simulink model "simplified_model"  (R2018b)
settings: Solver=VariableStepAuto  StartTime=0.0  StopTime=20  RelTol=1e-3
settings Model: Creator=dylan  LastModifiedBy=dylan

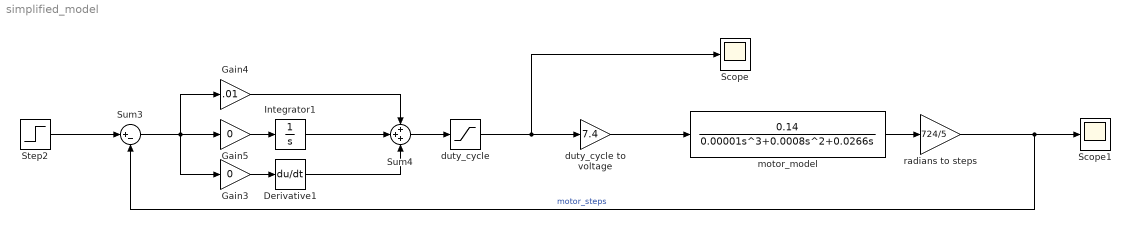
== system simplified_model ==
  Derivative1 : Derivative
  Gain3 : Gain  Gain=0
  Gain4 : Gain  Gain=.01
  Gain5 : Gain  Gain=0
  Integrator1 : Integrator
  Scope : Scope
  Scope1 : Scope
  Step2 : Step  After=1000  SampleTime=0
  Sum3 : Sum  Inputs=|+-
  Sum4 : Sum  Inputs=+++
  duty_cycle : Saturate  UpperLimit=1  LowerLimit=-1
  duty_cycle to voltage : Gain  Gain=7.4
  motor_model : TransferFcn  Numerator=[0.14]  Denominator=[0.00001 0.0008 0.0266 0]
  radians to steps : Gain  Gain=724/5
  wires:
  Integrator1/1 -> Sum4/2
  Gain4/1 -> Sum4/1
  Sum3/1 -> Gain3/1, Gain5/1, Gain4/1
  Gain5/1 -> Integrator1/1
  Derivative1/1 -> Sum4/3
  Step2/1 -> Sum3/1
  Gain3/1 -> Derivative1/1
  duty_cycle/1 -> duty_cycle to voltage/1, Scope/1
  motor_model/1 -> radians to steps/1
  Sum4/1 -> duty_cycle/1
  duty_cycle to voltage/1 -> motor_model/1
  radians to steps/1 -> Scope1/1, Sum3/2  "motor_steps"
